simulink model "mRobotArmControl"  (R2021a)
settings: Solver=FixedStepAuto  StartTime=0.0  StopTime=inf  RelTol=1e-3  EnableMultiTasking=on
InitFcn:
  | cBase=90;
  | cShoulder=90;
  | cElbow=90;
  | cWristVer=90;
  | cWristRot=90;
  | cGripper=73;
libraries: arduinolib x13
settings Model: SILPILModeSetting=veronly  ExtModeTrigDuration=2  Creator=loris  LastModifiedBy=angelo
settings OptimizationCC: EnhancedBackFolding=on  PassReuseOutputArgsAs=Individual arguments  ZeroExternalMemoryAtStartup=off  ZeroInternalMemoryAtStartup=off  MaxStackSize=64  OptimizeBlockOrder=speed  DifferentSizesBufferReuse=on  OptimizationCustomize=off  EfficientTunableParamExpr=on
settings DebuggingCC: ParameterTunabilityLossMsg=error
settings HardwareCC: ProdBitPerInt=16  ProdBitPerPointer=16  ProdBitPerSizeT=16  ProdBitPerPtrDiffT=16  ProdLargestAtomicFloat=None  ProdWordSize=8  ProdHWDeviceType=Atmel->AVR
settings SFSimCC: MATLABDynamicMemAlloc=off
settings RTWCC: SystemTargetFile=ert.tlc  HardwareBoard=Arduino Mega 2560  TemplateMakefile=ert_default_tmf  Toolchain=Arduino AVR  BuildConfiguration=Faster Runs
settings CodeAppCC: ForceParamTrailComments=on  IgnoreCustomStorageClasses=off  OperatorAnnotations=on  SimulinkDataObjDesc=on  SFDataObjDesc=on  InsertBlockDesc=on
settings ERTTargetCC: TargetLangStandard=C99 (ISO)  SupportContinuousTime=on  SupportVariableSizeSignals=on  ExtModeStaticAllocSize=2048  RootIOFormat=Structure reference

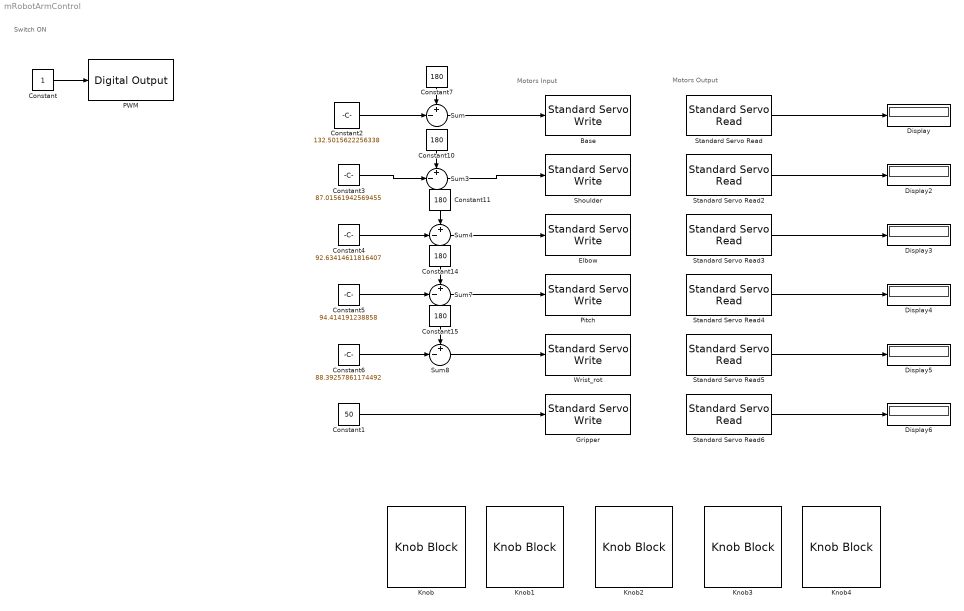
== system mRobotArmControl ==
  note: Motors Output
  note: Switch ON
  note: Motors Input
  Base : arduinolib/Standard Servo Write  pinNumber=11  ServoIndex=0  blockPlatform=ARDUINO
  Constant : Constant
  Constant1 : Constant  Value=50
  Constant{7,10..11,14..15} (5 alike) : Constant  Value=180
  Constant2 : Constant  Value=132.5015622256338
  Constant3 : Constant  Value=87.01561942569455
  Constant4 : Constant  Value=92.63414611816407
  Constant5 : Constant  Value=94.414191238858
  Constant6 : Constant  Value=88.39257861174492
  Display{,2..6} (6 alike) : Display
  Elbow : arduinolib/Standard Servo Write  pinNumber=9  ServoIndex=1  blockPlatform=ARDUINO
  Gripper : arduinolib/Standard Servo Write  pinNumber=3  ServoIndex=2  blockPlatform=ARDUINO
  Knob{,2..4} (4 alike) : KnobBlock  ScaleMax=180
  Knob1 : KnobBlock  ScaleMin=15  ScaleMax=165
  PWM : arduinolib/Digital Output  pinNumber=12  Direction=output  blockPlatform=arduino
  Pitch : arduinolib/Standard Servo Write  pinNumber=6  ServoIndex=3  blockPlatform=ARDUINO
  Shoulder : arduinolib/Standard Servo Write  pinNumber=10  ServoIndex=4  blockPlatform=ARDUINO
  Standard Servo Read : arduinolib/Standard Servo Read  pinNumber=11  SampleTime=0.1  ServoIndex=0  blockPlatform=ARDUINO
      settings: SourceProductBaseCode=ARDUINO
  Standard Servo Read2 : arduinolib/Standard Servo Read  pinNumber=10  SampleTime=0.1  ServoIndex=4  blockPlatform=ARDUINO
      settings: SourceProductBaseCode=ARDUINO
  Standard Servo Read3 : arduinolib/Standard Servo Read  pinNumber=9  SampleTime=0.1  ServoIndex=1  blockPlatform=ARDUINO
      settings: SourceProductBaseCode=ARDUINO
  Standard Servo Read4 : arduinolib/Standard Servo Read  pinNumber=6  SampleTime=0.1  ServoIndex=3  blockPlatform=ARDUINO
      settings: SourceProductBaseCode=ARDUINO
  Standard Servo Read5 : arduinolib/Standard Servo Read  pinNumber=5  SampleTime=0.1  ServoIndex=5  blockPlatform=ARDUINO
      settings: SourceProductBaseCode=ARDUINO
  Standard Servo Read6 : arduinolib/Standard Servo Read  pinNumber=3  SampleTime=0.1  ServoIndex=2  blockPlatform=ARDUINO
      settings: SourceProductBaseCode=ARDUINO
  Sum{,3..4,7..8} (5 alike) : Sum  Inputs=+-|
  Wrist_rot : arduinolib/Standard Servo Write  pinNumber=5  ServoIndex=5  blockPlatform=ARDUINO
  wires:
  Constant/1 -> PWM/1
  Sum/1 -> Base/1
  Constant2/1 -> Sum/2
  Constant7/1 -> Sum/1
  Constant1/1 -> Gripper/1
  Standard Servo Read6/1 -> Display6/1
  Constant10/1 -> Sum3/1
  Constant3/1 -> Sum3/2
  Sum3/1 -> Shoulder/1
  Constant11/1 -> Sum4/1
  Sum4/1 -> Elbow/1
  Constant4/1 -> Sum4/2
  Constant14/1 -> Sum7/1
  Sum7/1 -> Pitch/1
  Constant5/1 -> Sum7/2
  Constant15/1 -> Sum8/1
  Sum8/1 -> Wrist_rot/1
  Constant6/1 -> Sum8/2
  Standard Servo Read/1 -> Display/1
  Standard Servo Read2/1 -> Display2/1
  Standard Servo Read3/1 -> Display3/1
  Standard Servo Read4/1 -> Display4/1
  Standard Servo Read5/1 -> Display5/1
